simulink model "vehicle_prototype"  (R2024a)
settings: Solver=VariableStepAuto  StartTime=0.0  StopTime=inf  RelTol=1e-3
libraries: simulink x9
settings Model: Creator=admin  LastModifiedBy=admin

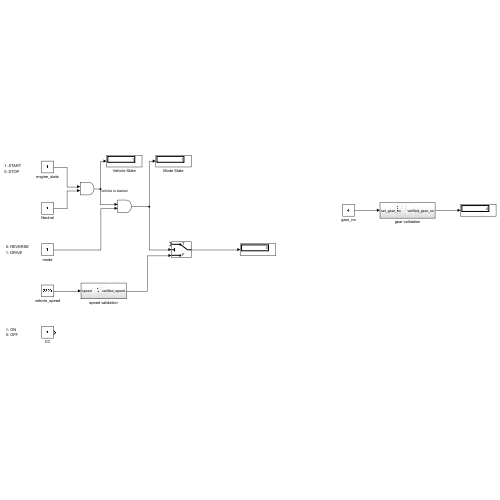
[thumbnail: Simulink's stored preview of the top-level diagram]
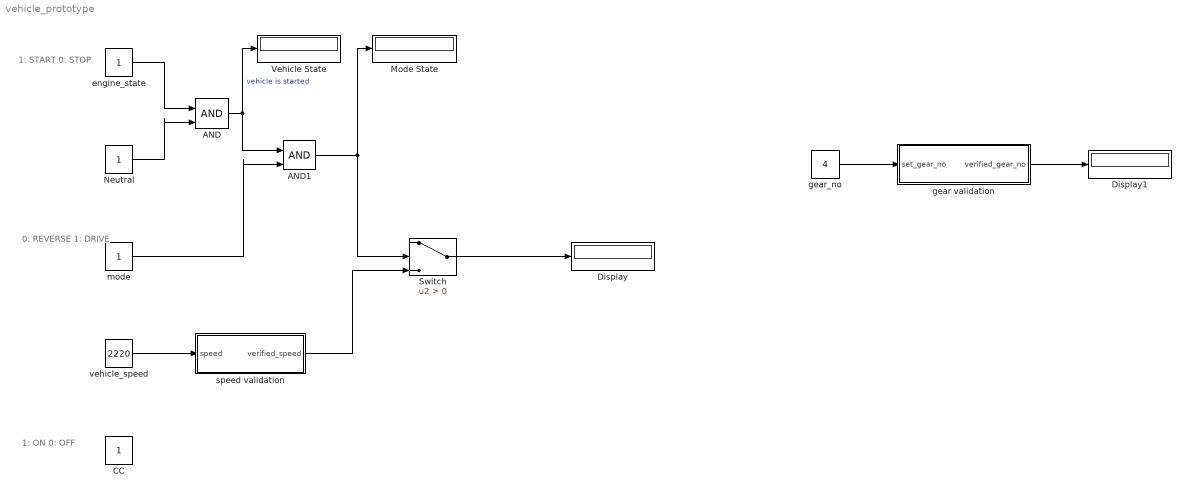
== system vehicle_prototype ==
  note: 0: REVERSE
      | 1: DRIVE
  note: 1: START
      | 0: STOP
  note: 1: ON
      | 0: OFF
  AND : Logic  IconShape=distinctive  AllPortsSameDT=off  OutDataTypeStr=boolean
  AND1 : Logic  IconShape=distinctive  AllPortsSameDT=off  OutDataTypeStr=boolean
  CC : Constant
  Display : Display
  Display1 : Display
  Mode State : Display
  Neutral : Constant
  Switch : Switch  Criteria=u2 > Threshold  SaturateOnIntegerOverflow=off  InputSameDT=off
  Vehicle State : Display
  engine_state : Constant
  gear validation : Subsystem
  gear_no : Constant  Value=4
  mode : Constant
  speed validation : Subsystem
  vehicle_speed : Constant  Value=2220
  wires:
  engine_state/1 -> AND/1
  Neutral/1 -> AND/2
  AND/1 -> AND1/1, Vehicle State/1  "vehicle is started"
  mode/1 -> AND1/2
  AND1/1 -> Switch/2, Mode State/1
  vehicle_speed/1 -> speed validation/1(speed)
  speed validation/1(verified_speed) -> Switch/3
  Switch/1 -> Display/1
  gear_no/1 -> gear validation/1(set_gear_no)
  gear validation/1(verified_gear_no) -> Display1/1

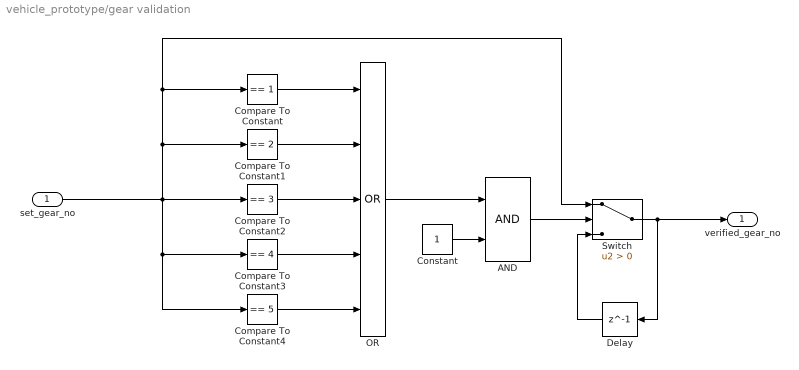
== system vehicle_prototype/gear validation ==
  set_gear_no : Inport
  AND : Logic  IconShape=distinctive  AllPortsSameDT=off  OutDataTypeStr=boolean
  Compare To Constant : simulink/Logic and Bit Operations/Compare To Constant  relop===  const=1  OutDataTypeStr=boolean
  Compare To Constant1 : simulink/Logic and Bit Operations/Compare To Constant  relop===  const=2  OutDataTypeStr=boolean
  Compare To Constant2 : simulink/Logic and Bit Operations/Compare To Constant  relop===  const=3  OutDataTypeStr=boolean
  Compare To Constant3 : simulink/Logic and Bit Operations/Compare To Constant  relop===  const=4  OutDataTypeStr=boolean
  Compare To Constant4 : simulink/Logic and Bit Operations/Compare To Constant  relop===  const=5  OutDataTypeStr=boolean
  Constant : Constant
  Delay : Delay  DelayLength=1  InitialCondition=1
  OR : Logic  Operator=OR  Inputs=5  IconShape=distinctive  AllPortsSameDT=off  OutDataTypeStr=boolean
  Switch : Switch  Criteria=u2 > Threshold  SaturateOnIntegerOverflow=off  InputSameDT=off
  verified_gear_no : Outport
  wires:
  set_gear_no/1 -> Compare To Constant3/1, Compare To Constant4/1, Compare To Constant2/1, Compare To Constant1/1, Switch/1, Compare To Constant/1
  Compare To Constant/1 -> OR/1
  Compare To Constant1/1 -> OR/2
  Compare To Constant2/1 -> OR/3
  Compare To Constant3/1 -> OR/4
  Compare To Constant4/1 -> OR/5
  OR/1 -> AND/1
  Constant/1 -> AND/2
  AND/1 -> Switch/2
  Switch/1 -> Delay/1, verified_gear_no/1
  Delay/1 -> Switch/3

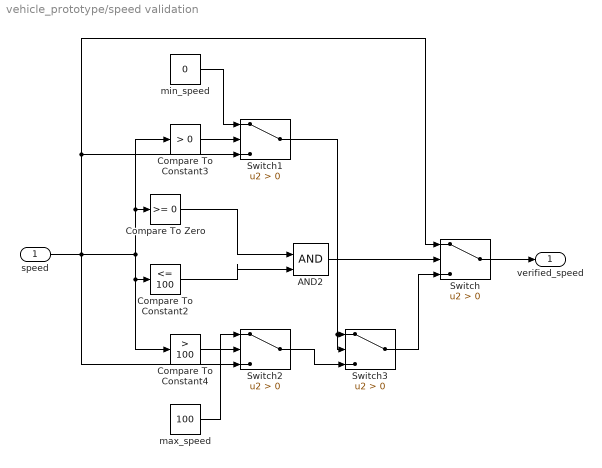
== system vehicle_prototype/speed validation ==
  speed : Inport
  AND2 : Logic  IconShape=distinctive  AllPortsSameDT=off  OutDataTypeStr=boolean
  Compare To Constant2 : simulink/Logic and Bit Operations/Compare To Constant  relop=<=  const=100  OutDataTypeStr=boolean
  Compare To Constant3 : simulink/Logic and Bit Operations/Compare To Constant  relop=>  const=0  OutDataTypeStr=boolean
  Compare To Constant4 : simulink/Logic and Bit Operations/Compare To Constant  relop=>  const=100  OutDataTypeStr=boolean
  Compare To Zero : simulink/Logic and Bit Operations/Compare To Zero  relop=>=  OutDataTypeStr=boolean
  Switch{,1..3} (4 alike) : Switch  Criteria=u2 > Threshold  SaturateOnIntegerOverflow=off  InputSameDT=off
  max_speed : Constant  Value=100
  min_speed : Constant  Value=0
  verified_speed : Outport
  wires:
  Compare To Constant4/1 -> Switch2/2
  AND2/1 -> Switch/2
  Switch3/1 -> Switch/3
  Compare To Zero/1 -> AND2/1
  min_speed/1 -> Switch1/1
  Switch2/1 -> Switch3/3
  Compare To Constant2/1 -> AND2/2
  max_speed/1 -> Switch2/1
  Compare To Constant3/1 -> Switch1/2
  Switch1/1 -> Switch3/1, Switch3/2
  speed/1 -> Switch2/3, Compare To Constant3/1, Compare To Zero/1, Compare To Constant4/1, Compare To Constant2/1, Switch/1, Switch1/3
  Switch/1 -> verified_speed/1
